simulink model "T37_SimulinkModel"  (R2023b)
settings: Solver=VariableStepAuto  StartTime=0.0  StopTime=10.0  RelTol=1e-3
values from neighbouring files (symbols this model uses):
  Fax = 0    [hw1.m]
  Fay = 0    [hw1.m]
  Faz = 0    [hw1.m]
  Ftx = 0    [hw1.m]
  Fty = 0    [hw1.m]
  Ftz = 0    [hw1.m]
  g = -9.81    [hw1.m]
  m = 0    [hw1.m]
  P = 1    [hw1.m]
  phi = 0    [hw1.m]
  psi = 0    [hw1.m]
  Q = 1    [hw1.m]
  R = 1    [hw1.m]
  theta = 0    [hw1.m]
  U = 1    [hw1.m]
  V = 1    [hw1.m]
  velocity = 100    [hw1.m]
  W = 1    [hw1.m]
settings Model: Creator=Owner  LastModifiedBy=Owner

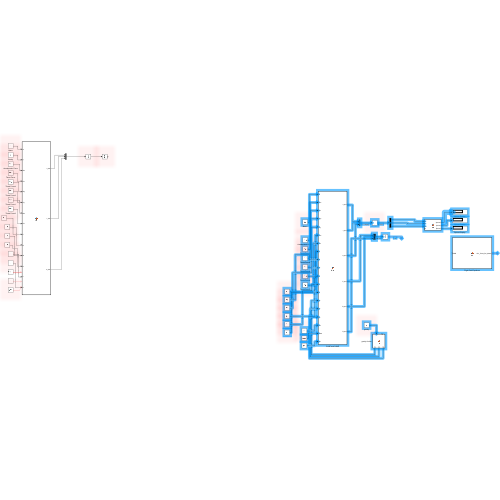
[thumbnail: Simulink's stored preview of the top-level diagram]
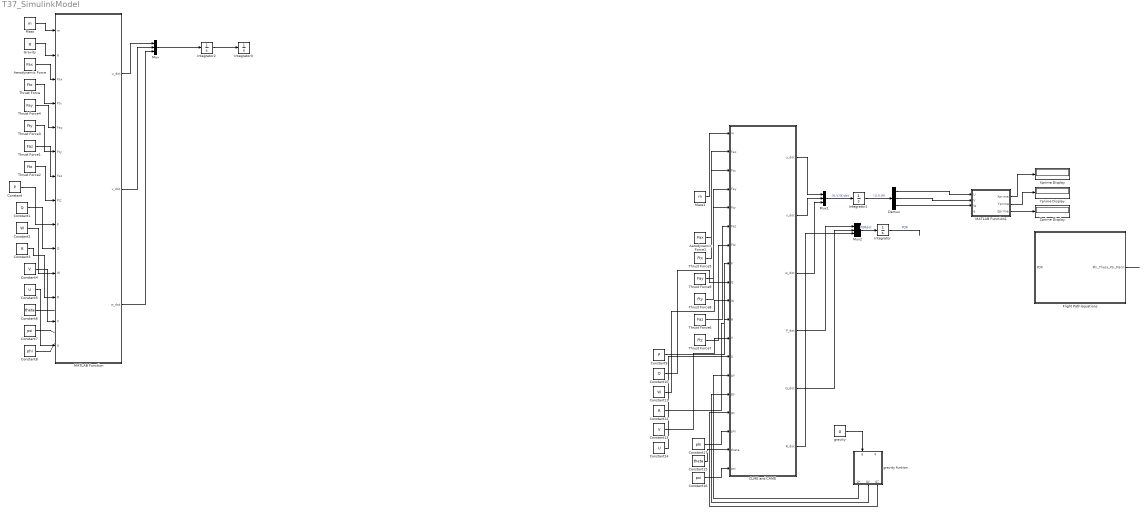
== system T37_SimulinkModel ==
  Aerodynamic Force : Constant  Value=Fax
  Aerodynamic Force1 : Constant  Value=Fax
  CLME and CAME : MATLAB Function  TreatAsAtomicUnit=on
  Constant : Constant  Value=P
  Constant1 : Constant  Value=Q
  Constant10 : Constant  Value=Q
  Constant11 : Constant  Value=W
  Constant12 : Constant  Value=R
  Constant13 : Constant  Value=V
  Constant14 : Constant  Value=U
  Constant15 : Constant  Value=theta
  Constant16 : Constant  Value=psi
  Constant17 : Constant  Value=phi
  Constant2 : Constant  Value=W
  Constant3 : Constant  Value=R
  Constant4 : Constant  Value=V
  Constant5 : Constant  Value=U
  Constant6 : Constant  Value=theta
  Constant7 : Constant  Value=psi
  Constant8 : Constant  Value=phi
  Constant9 : Constant  Value=P
  Demux : Demux  Outputs=3
  Flight Path Equations : MATLAB Function  TreatAsAtomicUnit=on
  Gravity : Constant  Value=g
  Integrator : Integrator
  Integrator1 : Integrator  InitialCondition=velocity
  Integrator2 : Integrator  InitialCondition=velocity
  Integrator3 : Integrator  InitialCondition=t
  MATLAB Function : MATLAB Function  TreatAsAtomicUnit=on
  MATLAB Function1 : MATLAB Function  TreatAsAtomicUnit=on
  Mass : Constant  Value=m
  Mass1 : Constant  Value=m
  Mux : Mux  Inputs=3
  Mux1 : Mux  Inputs=3
  Mux2 : Mux  Inputs=3
  Thrust Force : Constant  Value=Ftx
  Thrust Force1 : Constant  Value=Faz
  Thrust Force2 : Constant  Value=Ftz
  Thrust Force3 : Constant  Value=Fty
  Thrust Force4 : Constant  Value=Fay
  Thrust Force5 : Constant  Value=Ftx
  Thrust Force6 : Constant  Value=Faz
  Thrust Force7 : Constant  Value=Ftz
  Thrust Force8 : Constant  Value=Fty
  Thrust Force9 : Constant  Value=Fay
  Xprime Display : Display
  Yprime Display : Display
  Zprime Display : Display
  gravity : Constant  Value=g
  gravity funtion : MATLAB Function  TreatAsAtomicUnit=on
  wires:
  MATLAB Function/1(u_dot) -> Mux/1
  Aerodynamic Force/1 -> MATLAB Function/3(Fax)
  Mass/1 -> MATLAB Function/1(m)
  Integrator2/1 -> Integrator3/1
  MATLAB Function/2(v_dot) -> Mux/2
  MATLAB Function/3(w_dot) -> Mux/3
  Mux/1 -> Integrator2/1
  Thrust Force/1 -> MATLAB Function/4(Ftx)
  Gravity/1 -> MATLAB Function/2(g)
  Constant/1 -> MATLAB Function/9(P)
  Constant1/1 -> MATLAB Function/10(Q)
  Constant2/1 -> MATLAB Function/11(W)
  Constant3/1 -> MATLAB Function/12(R)
  Constant4/1 -> MATLAB Function/13(V)
  Constant5/1 -> MATLAB Function/14(U)
  Thrust Force3/1 -> MATLAB Function/6(Fty)
  Thrust Force4/1 -> MATLAB Function/5(Fay)
  Thrust Force1/1 -> MATLAB Function/7(Faz)
  Thrust Force2/1 -> MATLAB Function/8(Ftz)
  Constant6/1 -> ?
  Constant7/1 -> ?
  Constant8/1 -> ?
  Integrator/1 -> ?  "PQR"
  Flight Path Equations/1(Phi_Theta_Psi_Matrix) -> ?
  Constant11/1 -> CLME and CAME/10(W)
  Thrust Force9/1 -> CLME and CAME/4(Fay)
  MATLAB Function1/3(Zprime) -> Zprime Display/1
  CLME and CAME/5(Q_dot) -> Mux2/2
  Constant16/1 -> CLME and CAME/19(psi)
  Aerodynamic Force1/1 -> CLME and CAME/2(Fax)
  Integrator1/1 -> Demux/1  "(U,V,W)"
  Constant10/1 -> CLME and CAME/9(Q)
  Mux1/1 -> Integrator1/1  "(U,V,W)dot"
  Demux/3 -> MATLAB Function1/3(W)
  Demux/2 -> MATLAB Function1/2(V)
  gravity funtion/3(gz) -> CLME and CAME/16(gz)
  CLME and CAME/6(R_dot) -> Mux2/3
  Thrust Force8/1 -> CLME and CAME/5(Fty)
  gravity funtion/2(gy) -> CLME and CAME/15(gy)
  Constant17/1 -> CLME and CAME/17(phi)
  Demux/1 -> MATLAB Function1/1(U)
  CLME and CAME/4(P_dot) -> Mux2/1
  gravity funtion/1(gx) -> CLME and CAME/14(gx)
  Mux2/1 -> Integrator/1  "PQRdot"
  MATLAB Function1/2(Yprime) -> Yprime Display/1
  Thrust Force7/1 -> CLME and CAME/7(Ftz)
  Mass1/1 -> CLME and CAME/1(m)
  Constant9/1 -> CLME and CAME/8(P)
  Thrust Force6/1 -> CLME and CAME/6(Faz)
  Constant14/1 -> CLME and CAME/13(U)
  Thrust Force5/1 -> CLME and CAME/3(Ftx)
  gravity/1 -> gravity funtion/1(g)
  Constant12/1 -> CLME and CAME/11(R)
  CLME and CAME/2(v_dot) -> Mux1/2
  Constant13/1 -> CLME and CAME/12(V)
  CLME and CAME/1(u_dot) -> Mux1/1
  Constant15/1 -> CLME and CAME/18(theta)
  CLME and CAME/3(w_dot) -> Mux1/3
  MATLAB Function1/1(Xprime) -> Xprime Display/1

== matlab function T37_SimulinkModel/gravity funtion ==
  data: g input; gx output; gy output; gz output; q input
function [gx, gy, gz] = fcn(g,q)

gx = -gsind(q(1,:));
gy = g*((cosd(q(2,:))).*(sind(q(2,:))));
gz = g*((cosd(3,:)).*(cosd(3,:)));


%function [gx, gy, gz] = fcn(g,phi, theta, psi)

%gx = -gsind(theta);
%gy = g*((cosd(theta)).*(sind(phi)));
%gz = g*((cosd(theta)).*(cosd(phi)));

== matlab function T37_SimulinkModel/CLME and CAME ==
  data: m input; Fax input; Ftx input; Fay input; Fty input; Faz input; Ftz input; P input; Q input; W input; R input; V input; U input; u_dot output; gx input; v_dot output; w_dot output; P_dot output; Q_dot output; R_dot output; gy input; gz input; phi input; theta input; psi input
function [u_dot, v_dot, w_dot, P_dot, Q_dot, R_dot] = fcn(m, Fax, Ftx, Fay, Fty, Faz, Ftz, P, Q, W, R, V, U, gx, gy, gz, phi, theta, psi)

%Mass = 2300; %kg
%g = 9.81; %m/s
%theta = 0;
%Fax = 0;
%Ftx = 0;


u_dot = (1/m) * (((m*gx)+ (Fax + Ftx))-(Q*W)+(R*V));
v_dot = (1/m) * (((m*gy)+ (Fay + Fty))-(U*R)+(P*W));
w_dot = (1/m) * (((m*gz)+ (Faz + Ftz))-(P*V)+(Q*U));



%CAME
%Ixx=[];
%Ixz=[];
%Izz=[];
%Iyy=[];
%La=0;
%Lt=0;
%Ma=0;
%Mt=0;
%Na=0;
%Nt=0;


R_dot = ((Na+Nt)+(P.*Ixz)-((P.*Q).*(Iyy-Ixx))-((Q.*R).*Ixz))./(Izz);
P_dot = ((La+Lt)+(R_dot.*Ixz)+(P.*Q.*Ixz)-(R*Q).*(Izz-Iyy))./(Ixx); %need to change so that Pdot is taken into account - page 408/409 of the one grad paper - Calmoon
Q_dot = ((Ma+Mt)-(R_dot.*Ixz)+(P.*Q.*Ixz)-(R*Q).*(Izz-Iyy))./(Iyy);

== matlab function T37_SimulinkModel/MATLAB Function ==
  data: m input; u_dot output; g input; Fax input; v_dot output; w_dot output; Ftx input; Fay input; Fty input; Faz input; Ftz input; P input; Q input; W input; R input; V input; U input
function [u_dot, v_dot, w_dot] = fcn(m, g, Fax, Ftx, Fay, Fty, Faz, Ftz, P, Q, W, R, V, U)

%Mass = 2300; %kg
%g = 9.81; %m/s
%theta = 0;
%Fax = 0;
%Ftx = 0;


u_dot = (1/m) * (((m*g)+ (Fax + Ftx))-(Q*W)+(R*V));
v_dot = (1/m) * (((m*g)+ (Fay + Fty))-(U*R)+(P*W));
w_dot = (1/m) * (((m*g)+ (Faz + Ftz))-(P*V)+(Q*U));



%CAME
%Ixx=[];
%Ixz=[];
%Izz=[];
%Iyy=[];
%La=0;
%Lt=0;
%Ma=0;
%Mt=0;
%Na=0;
%Nt=0;



%P_dot = ((La+Lt)+(R_dot.*Ixz)+(P.*Q.*Ixz)-(R*Q).*(Izz-Iyy))./(Ixx)
%Q_dot = ((Ma+Mt)-(R_dot.*Ixz)+(P.*Q.*Ixz)-(R*Q).*(Izz-Iyy))./(Iyy

== matlab function T37_SimulinkModel/Flight Path Equations ==
  data: PQR input; Phi_Theta_Psi_Matrix output
function Phi_Theta_Psi_Matrix = fcn(PQR)

AngleMatrix = [1 (sind(phi)).*(tand(theta)) ((cosd(phi)).*tand(theta));
               0 cosd(phi) -sind(phi); 
               0 ((sind(phi)).*(secd(theta))) ((cosd(phi)).*(secd(theta)))]; 

%check if actually a cross product

Phi_Theta_Psi_Matrix = cross(AngleMatrix, PQR);

== matlab function T37_SimulinkModel/MATLAB Function1 ==
  data: U input; Xprime output; V input; W input; Yprime output; Zprime output; q input
function [Xprime, Yprime, Zprime] = fcn(U, V, W, q)
%function [Xprime, Yprime, Zprime] = fcn(U, V, W, phi, theta, psi)
%need to take angles out and replace with quaternions

%RotationMatrix = [cosd(psi).*cosd(theta) (-sind(psi).*cosd(phi))+(cosd(psi).*(sind(theta)).*sind(phi)) ((sind(psi).*sind(phi))+(cosd(psi).*(sind(theta)).*cosd(phi)));
                 % (sind(psi) .* cosd(theta)) (cosd(psi) .* cosd(phi))+(sind(phi).*sind(theta) .* sind(phi)) -(sind(phi).*(cosd(psi)))+(sind(psi).*(sind(theta)).*(cosd(phi)))
                 % (-sind(theta)) (cosd(theta).*(sind(phi))) ((cosd(theta)) .* cosd(phi))];

%replace phi, theta, psi with q1,q2,q3
qMatrix = RotationMatrix(q);

%Xprime = U.*RotationMatrix(1,:);
%Yprime = V.*(RotationMatrix(2,:));
%Zprime = W .*(RotationMatrix(3,:));

Xprime = U.*qMatrix;
Yprime = V.*qMatrix;
Zprime = W .*qMatrix;
